simulink model "kindyn"  (R2019a)
settings: Solver=ode45  StartTime=0.0  StopTime=100  RelTol=1e-3  EnableMultiTasking=on
undefined symbols (not defined in the file): drawAircraft, plane_states, plotvtolstatevariables
libraries: simulink x6
settings Model: NumberOfSteps=1000  Creator=beard  LastModifiedBy=VTOL_HYD
settings DataIOCC: LimitDataPoints=on  SaveFormat=Array  SignalLoggingSaveFormat=ModelDataLogs  ReturnWorkspaceOutputs=off
settings OptimizationCC: ExpressionDepthLimit=2147483647  InitFltsAndDblsToZero=on  LifeSpan=inf
settings DebuggingCC: UnderspecifiedInitializationDetection=Classic  MergeDetectMultiDrivingBlocksExec=none  SolverPrmCheckMsg=warning  FcnCallInpInsideContextMsg=warning  AllowSymbolicDim=off  StateNameClashWarn=warning  PregeneratedLibrarySubsystemCodeDiagnostic=none  SFUnexpectedBacktrackingDiag=warning  SFNoUnconditionalDefaultTransitionDiag=warning  SFExecutionAtInitializationDiag=none  ArithmeticOperatorsInVariantConditions=warning
settings HardwareCC: ProdBitPerPointer=32  ProdBitPerSizeT=32  ProdBitPerPtrDiffT=32  ProdLargestAtomicFloat=None  ProdIntDivRoundTo=Undefined  ProdEndianess=Unspecified  ProdWordSize=32  ProdHWDeviceType=32-bit Generic
settings ModelReferenceCC: PropagateSignalLabelsOutOfModel=off
settings SFSimCC: SimUseLocalCustomCode=off
settings RTWCC: RTWUseLocalCustomCode=off
settings CodeAppCC: StateflowObjectComments=on
settings GRTTargetCC: TargetLangStandard=C89/C90 (ANSI)  GeneratePreprocessorConditionals=Disable all  CombineOutputUpdateFcns=off  GRTInterface=on
settings ConfigComp: CovMetricSettings=dw  CovHtmlReporting=on  CovSaveCumulativeToWorkspaceVar=on  CovSaveSingleToWorkspaceVar=on  CovExternalEMLEnable=off  CovSFcnEnable=off

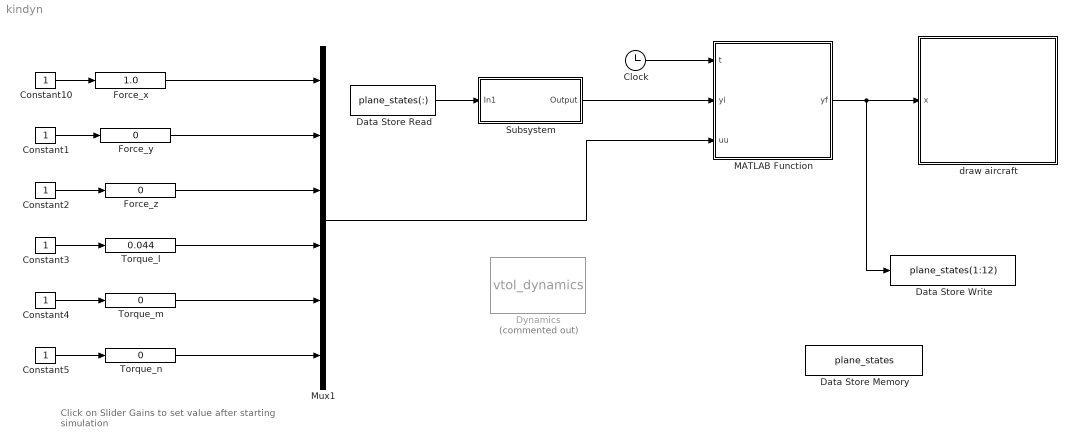
== system kindyn ==
  note: Click on Slider Gains to set value
      | after starting simulation
  Clock : Clock
  Constant{1..5,10} (6 alike) : Constant
  Data Store Memory : DataStoreMemory  DataStoreName=plane_states  ReadBeforeWriteMsg=warning  WriteAfterWriteMsg=warning  WriteAfterReadMsg=warning  InitialValue=[0;0;0;0;0;0;0;0;0;0;0;0]  ShowAdditionalParam=off
  Data Store Read : DataStoreRead  DataStoreName=plane_states  DataStoreElements=plane_states(:)
  Data Store Write : DataStoreWrite  DataStoreName=plane_states  DataStoreElements=plane_states(1:12)
  Dynamics : S-Function  Commented=on  FunctionName=vtol_dynamics  Parameters=vtol  SFunctionDeploymentMode=off  EnableBusSupport=off
  Force_x : simulink/Math Operations/Slider Gain  gain=1.0  low=-1  high=1
  Force_y : simulink/Math Operations/Slider Gain  gain=0  low=-1  high=1
  Force_z : simulink/Math Operations/Slider Gain  gain=0  low=-1  high=1
  MATLAB Function : MATLAB Function  InitFcn=|  TreatAsAtomicUnit=on
      | path(pathdef)
      | addpath('.')
  Mux1 : Mux  Inputs=6
  Subsystem : Subsystem  InitFcn=|
      | clear all
      | path(pathdef)
      | addpath('.')
  Torque_l : simulink/Math Operations/Slider Gain  gain=0.044  low=-0.1  high=0.1
  Torque_m : simulink/Math Operations/Slider Gain  gain=0  low=-0.1  high=0.1
  "Torque_n " : simulink/Math Operations/Slider Gain  gain=0  low=-0.1  high=0.1
  draw aircraft : Subsystem  InitFcn=|
      | path(pathdef)
      | addpath('.')
      mask Display: image(imread('../2_coord_frm/vtol.jpeg'))
  wires:
  Constant5/1 -> "Torque_n "/1
  Constant10/1 -> Force_x/1
  Constant1/1 -> Force_y/1
  Constant2/1 -> Force_z/1
  MATLAB Function/1(yf) -> Data Store Write/1, draw aircraft/1(x)
  Force_z/1 -> Mux1/3
  Force_y/1 -> Mux1/2
  Force_x/1 -> Mux1/1
  "Torque_n "/1 -> Mux1/6
  Constant4/1 -> Torque_m/1
  Torque_m/1 -> Mux1/5
  Constant3/1 -> Torque_l/1
  Torque_l/1 -> Mux1/4
  Clock/1 -> MATLAB Function/1(t)
  Mux1/1 -> MATLAB Function/3(uu)
  Subsystem/1(Output) -> MATLAB Function/2(yi)
  Data Store Read/1 -> Subsystem/1(In1)

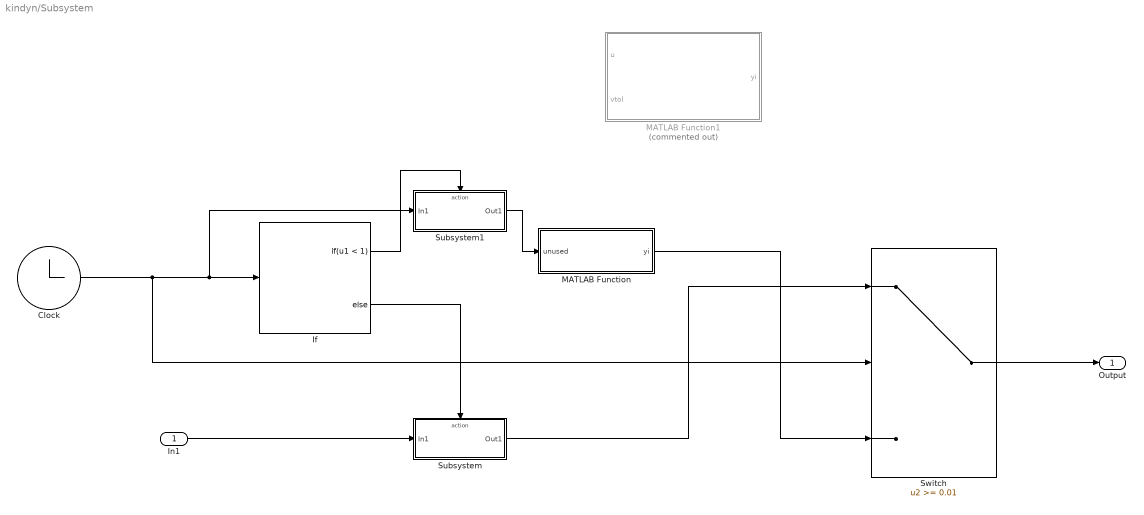
== system kindyn/Subsystem ==
  In1 : Inport
  Clock : Clock
  If : If  IfExpression=u1 < 1
  MATLAB Function : MATLAB Function  TreatAsAtomicUnit=on
  MATLAB Function1 : MATLAB Function  Commented=on  InitFcn=|  TreatAsAtomicUnit=on
      | path(pathdef)
      | addpath('.')
  Subsystem : Subsystem
  Subsystem1 : Subsystem
  Switch : Switch  Threshold=0.01
  Output : Outport
  wires:
  Clock/1 -> Switch/2, Subsystem1/1(In1), If/1
  If/2 -> Subsystem/Action
  In1/1 -> Subsystem/1(In1)
  Switch/1 -> Output/1
  Subsystem/1(Out1) -> Switch/1
  MATLAB Function/1(yi) -> Switch/3
  If/1 -> Subsystem1/Action
  Subsystem1/1(Out1) -> MATLAB Function/1(unused)

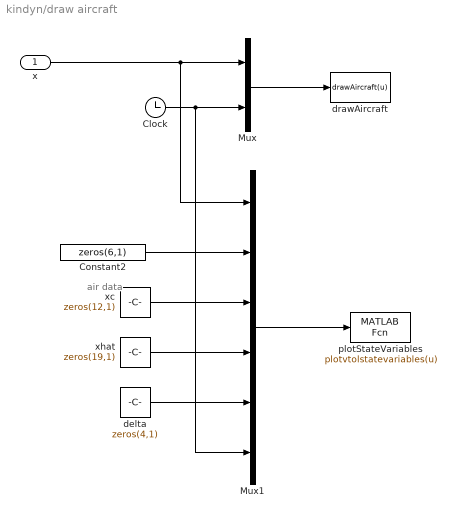
== system kindyn/draw aircraft ==
  note: air data
  x : Inport
  Clock : Clock
  Constant2 : Constant  Value=zeros(6,1)
  Mux : Mux  Inputs=2
  Mux1 : Mux  Inputs=6
  delta : Constant  Value=zeros(4,1)
  drawAircraft : MATLABFcn  MATLABFcn=drawAircraft(u)  OutputDimensions=0  SampleTime=0.1
  plotStateVariables : MATLABFcn  MATLABFcn=plotvtolstatevariables(u)  OutputDimensions=0  SampleTime=0.1
  xc : Constant  Value=zeros(12,1)
  xhat : Constant  Value=zeros(19,1)
  wires:
  Mux/1 -> drawAircraft/1
  x/1 -> Mux/1, Mux1/1
  Clock/1 -> Mux/2, Mux1/6
  Mux1/1 -> plotStateVariables/1
  xhat/1 -> Mux1/4
  xc/1 -> Mux1/3
  delta/1 -> Mux1/5
  Constant2/1 -> Mux1/2

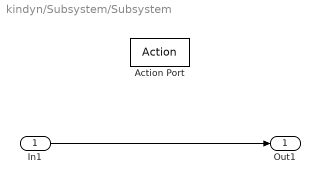
== system kindyn/Subsystem/Subsystem ==
  In1 : Inport
  Action Port : ActionPort  ActionPortLabel=else
  Out1 : Outport
  wires:
  In1/1 -> Out1/1

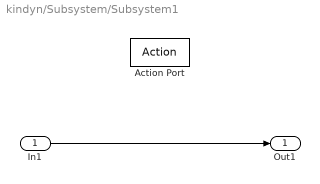
== system kindyn/Subsystem/Subsystem1 ==
  In1 : Inport
  Action Port : ActionPort  ActionPortLabel=if(u1 < 1)
  Out1 : Outport
  wires:
  In1/1 -> Out1/1

== matlab function kindyn/Subsystem/MATLAB Function1 ==
  data: u input; yi output; vtol input
function yi = init_states(u, vtol)
   
    yi(1)    = vtol.pn0;...
    yi(2)    = vtol.pe0;...
    yi(3)    = vtol.pd0;...
    yi(4)    = vtol.u0;...
    yi(5)    = vtol.v0;...
    yi(6)    = vtol.w0;...
    yi(7)    = vtol.phi0;...
    yi(8)    = vtol.theta0;...
    yi(9)    = vtol.psi0;...
    yi(10)   = vtol.p0;...
    yi(11)   = vtol.q0;...
    yi(12)   = vtol.r0;...
end

== matlab function kindyn/MATLAB Function ==
  data: t input; yf output; yi input; uu input
function yf = vtol_dynamics(t,yi,uu)

% vtol = vtol_parameters();
 

h = 0.01;

    pn    = yi(1);
    pe    = yi(2);
    pd    = yi(3);
    u     = yi(4);
    v     = yi(5);
    w     = yi(6);
    phi   = yi(7);
    theta = yi(8);
    psi   = yi(9);
    p     = yi(10);
    q     = yi(11);
    r     = yi(12);
    
    yi = [pn; pe; pd; u; v; w; phi; theta; psi; p; q; r];

% if t <= 0.005
%     
%     yf = [0,0,0,0,0,0,0,0,0,0,0,0]';
%     
% end
% fprintf('size of yi = %d\n', size(yi));
yf = zeros(12,1);

yf = rk4(t,yi,uu,h);

% fprintf('size of yi = %d\n', size(yi));

end

== matlab function kindyn/Subsystem/MATLAB Function ==
  data: yi output double; unused input
% initialize the VTOL viewer
function yi = vtol_parameters(~)

% addpath('../1_dependencies/tools');  
	% initial conditions
% 	vtol.pn0    = 0;     % initial North position
% 	vtol.pe0    = 0;     % initial East position
% 	vtol.pd0    = -200;  % initial Down position (negative altitude)
% 	vtol.u0     = [0.0582940477613936];     % initial velocity along body x-axis
% 	vtol.v0     = [1.50144609751618];     % initial velocity along body y-axis
% 	vtol.w0     = [7.75240280716845];     % initial velocity along body z-axis
% 	vtol.phi0   = [1.49323701803359];     % initial roll angle
% 	vtol.theta0 = [1.54331914556610];     % initial pitch angle
% 	vtol.psi0   = [1.50056503685554e-09];     % initial yaw angle
% 	e = Euler2Quaternion(vtol.phi0, vtol.theta0, vtol.psi0);
% 	vtol.e0     = e(1);  % initial quaternion
% 	vtol.e1     = e(2);
% 	vtol.e2     = e(3);
% 	vtol.e3     = e(4);
% 	vtol.p0     = [-9.99618859834988e-10];     % initial body frame roll rate
% 	vtol.q0     = [3.00308152458690e-11];     % initial body frame pitch rate
% 	vtol.r0     = [6.37914729992034e-12];     % initial body frame yaw rate
    
    vtol.pn0    = 0;     % initial North position
	vtol.pe0    = 0;     % initial East position
	vtol.pd0    = 0;  % initial Down position (negative altitude)
	vtol.u0     = 0;     % initial velocity along body x-axis
	vtol.v0     = 0;     % initial velocity along body y-axis
	vtol.w0     = 0;     % initial velocity along body z-axis
	vtol.phi0   = 0;     % initial roll angle
	vtol.theta0 = 0;     % initial pitch angle
	vtol.psi0   = 0;     % initial yaw angle
% 	e = Euler2Quaternion(vtol.phi0,vtol.theta0,vtol.psi0);
% 	vtol.e0     = e(1);  % initial quaternion
% 	vtol.e1     = e(2);
% 	vtol.e2     = e(3);
% 	vtol.e3     = e(4);
	vtol.p0     = 0;     % initial body frame roll rate
	vtol.q0     = 0;     % initial body frame pitch rate
	vtol.r0     = 0;     % initial body frame yaw rate
    
    yi = [0;0;0;0;0;0;0;0;0;0;0;0];
    
    yi(1)    = vtol.pn0;...
    yi(2)    = vtol.pe0;...
    yi(3)    = vtol.pd0;...
    yi(4)    = vtol.u0;...
    yi(5)    = vtol.v0;...
    yi(6)    = vtol.w0;...
    yi(7)    = vtol.phi0;...
    yi(8)    = vtol.theta0;...
    yi(9)    = vtol.psi0;...
    yi(10)   = vtol.p0;...
    yi(11)   = vtol.q0;...
    yi(12)   = vtol.r0;...

	   
% 	%physical parameters of airframe
% 	vtol.gravity = 9.81;
% 	vtol.mass = 13.5;
% 	vtol.Jx   = 0.8244;
% 	vtol.Jy   = 1.135;
% 	vtol.Jz   = 1.759;
% 	vtol.Jxz  = 0.1204;
% 	vtol.S_wing        = 0.55;
% 	vtol.b             = 2.90;
% 	vtol.c             = 0.19;
% 	vtol.S_prop        = 0.2027;
% 	vtol.rho           = 1.2682;
% 	vtol.e             = 0.9;
% %  	vtol.AR            = vtol.b^2/vtol.S_wing;
% 
% 	% Gamma parameters 
% % 	vtol.Gamma  = vtol.Jx*vtol.Jz-vtol.Jxz^2;
% % 	vtol.Gamma1 = (vtol.Jxz*(vtol.Jx-vtol.Jy+vtol.Jz))/vtol.Gamma;
% % 	vtol.Gamma2 = (vtol.Jz*(vtol.Jz-vtol.Jy)+vtol.Jxz*vtol.Jxz)/vtol.Gamma;
% % 	vtol.Gamma3 = vtol.Jz/vtol.Gamma;
% % 	vtol.Gamma4 = vtol.Jxz/vtol.Gamma;
% % 	vtol.Gamma5 = (vtol.Jz-vtol.Jx)/vtol.Jy;
% % 	vtol.Gamma6 = vtol.Jxz/vtol.Jy;
% % 	vtol.Gamma7 = (vtol.Jx*(vtol.Jx-vtol.Jy)+vtol.Jxz*vtol.Jxz)/vtol.Gamma;
% % 	vtol.Gamma8 = vtol.Jx/vtol.Gamma;
% 
% 	%%%%%%%%%%%%%%%%%%%%%%%%%%%%%%%%%
% 	% aerodynamic coefficients
% 	vtol.C_L_0         = 0.28;
% 	vtol.C_D_0         = 0.03;
% 	vtol.C_m_0         = -0.02338;
% 	vtol.C_L_alpha     = 3.45;
% 	vtol.C_D_alpha     = 0.30;
% 	vtol.C_m_alpha     = -0.38;
% 	vtol.C_L_q         = 0;
% 	vtol.C_D_q         = 0.0;
% 	vtol.C_m_q         = -3.6;
% 	vtol.C_L_delta_e   = -0.36;
% 	vtol.C_D_delta_e   = 0.0;
% 	vtol.C_m_delta_e   = -0.5;
% 	vtol.M             = 50;
% 	vtol.alpha0        = 0.4712;
% 	vtol.epsilon       = 0.16;
% 	vtol.C_D_p         = 0.0437;
% 
% 	vtol.C_Y_0         = 0.0;
% 	vtol.C_ell_0       = 0.0;
% 	vtol.C_n_0         = 0.0;
% 	vtol.C_Y_beta      = -0.98;
% 	vtol.C_ell_beta    = -0.12;
% 	vtol.C_n_beta      = 0.25;
% 	vtol.C_Y_p         = 0.0;
% 	vtol.C_ell_p       = -0.26;
% 	vtol.C_n_p         = 0.022;
% 	vtol.C_Y_r         = 0.0;
% 	vtol.C_ell_r       = 0.14;
% 	vtol.C_n_r         = -0.35;
% 	vtol.C_Y_delta_a   = 0.0;
% 	vtol.C_ell_delta_a = 0.08;
% 	vtol.C_n_delta_a   = 0.06;
% 	vtol.C_Y_delta_r   = -0.17;
% 	vtol.C_ell_delta_r = 0.105;
% 	vtol.C_n_delta_r   = -0.032;
% 
% 	% Parameters for propulsion thrust and torque models
% 	vtol.D_prop = 0.508;     % prop diameter in m
% 
% 	% Motor parameters
% 	vtol.K_V = 145;                    % from datasheet RPM/V
% % 	vtol.KQ = (1/vtol.K_V)*60/(2*pi);   % KQ in N-m/A, V-s/rad
% % 	vtol.R_motor = 0.042;              % ohms
% % 	vtol.i0 = 1.5;                     % no-load (zero-torque) current (A)
% % 
% % 	% Inputs
% % 	vtol.ncells = 12;
% % 	vtol.V_max = 3.7*vtol.ncells;       % max voltage for specified number of battery cells
% % 
% % 	% Coeffiecients from prop_data fit
% % 	vtol.C_Q2 = -0.01664;
% % 	vtol.C_Q1 = 0.004970;
% % 	vtol.C_Q0 = 0.005230;
% % 
% % 	vtol.C_T2 = -0.1079;
% % 	vtol.C_T1 = -0.06044;
% % 	vtol.C_T0 = 0.09357;
end
